simulink model "DNNCells_tSPMeA_BatteryPack_Passive100cellBal_RestCycler"  (R2024a)
settings: Solver=VariableStepAuto  StartTime=0.0  StopTime=1E7  RelTol=1e-3
undefined symbols (not defined in the file or in its folder): battery_builder_rtmsupport, gcbh
libraries: fl_lib x38, nesl_utility x36, simulink x26, BatteryLibrary_lib x6
(part 2 of 2)

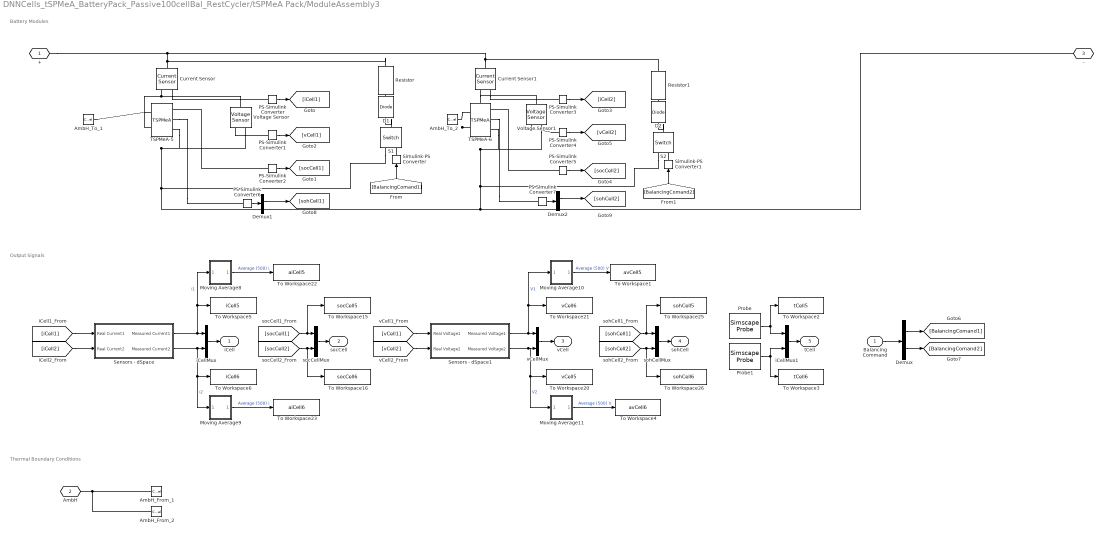
== system DNNCells_tSPMeA_BatteryPack_Passive100cellBal_RestCycler/tSPMeA Pack/ModuleAssembly3 ==
  note: Battery Modules
  note: Thermal Boundary Conditions
  note: Output Signals
  Balancing Command : Inport
  AmbH_From_1 : ConnectionLabel  Label=ambH_1
  AmbH_From_2 : ConnectionLabel  Label=ambH_2
  AmbH_To_1 : ConnectionLabel  Label=ambH_1
  AmbH_To_2 : ConnectionLabel  Label=ambH_2
  Current Sensor : fl_lib/Electrical/Electrical Sensors/Current Sensor
  Current Sensor1 : fl_lib/Electrical/Electrical Sensors/Current Sensor
  D1 : fl_lib/Electrical/Electrical Elements/Diode  Vf=0.6 V  Ron=0.3 Ohm  Goff=1e-8 1/Ohm  i_specify=off  i_priority=None  i=0 A  i_nominal_specify=off  i_nominal_value=1  i_nominal_unit=A  v_specify=off  v_priority=None  v=0 V  v_nominal_specify=off  v_nominal_value=1  v_nominal_unit=V
      settings: LogSimulationData=on
  D2 : fl_lib/Electrical/Electrical Elements/Diode  Vf=0.6 V  Ron=0.3 Ohm  Goff=1e-8 1/Ohm  i_specify=off  i_priority=None  i=0 A  i_nominal_specify=off  i_nominal_value=1  i_nominal_unit=A  v_specify=off  v_priority=None  v=0 V  v_nominal_specify=off  v_nominal_value=1  v_nominal_unit=V
      settings: LogSimulationData=on
  Demux : Demux  Outputs=2
  Demux1 : Demux
  Demux2 : Demux
  Moving Average10 : Subsystem
  Moving Average11 : Subsystem
  Moving Average8 : Subsystem
  Moving Average9 : Subsystem
  PS-Simulink Converter{,1..7} (8 alike) : nesl_utility/PS-Simulink Converter  PhysicalDomain=network_engine_domain  SubClassName=ps_output  LeftPortType=input  RightPortType=output  PseudoPeriodic=off  Frequencies=[]  VectorFormat=inherit  Unit=inherit  AffineConversion=off
  Probe : SimscapeProbe  BoundBlock=426  Variables={T}
  Probe1 : SimscapeProbe  BoundBlock=427  Variables={T}
  Resistor : fl_lib/Electrical/Electrical Elements/Resistor  R=0.001 Ohm  i_specify=off  i_priority=None  i=0 A  i_nominal_specify=off  i_nominal_value=1  i_nominal_unit=A  v_specify=off  v_priority=None  v=0 V  v_nominal_specify=off  v_nominal_value=1  v_nominal_unit=V
  Resistor1 : fl_lib/Electrical/Electrical Elements/Resistor  R=0.001 Ohm  i_specify=off  i_priority=None  i=0 A  i_nominal_specify=off  i_nominal_value=1  i_nominal_unit=A  v_specify=off  v_priority=None  v=0 V  v_nominal_specify=off  v_nominal_value=1  v_nominal_unit=V
  S1 : fl_lib/Electrical/Electrical Elements/Switch  R_closed=0.01 Ohm  G_open=1e-8 1/Ohm  Threshold=0.5  i_specify=off  i_priority=None  i=0 A  i_nominal_specify=off  i_nominal_value=1  i_nominal_unit=A  v_specify=off  v_priority=None  v=0 V  v_nominal_specify=off  v_nominal_value=1  v_nominal_unit=V
  S2 : fl_lib/Electrical/Electrical Elements/Switch  R_closed=0.01 Ohm  G_open=1e-8 1/Ohm  Threshold=0.5  i_specify=off  i_priority=None  i=0 A  i_nominal_specify=off  i_nominal_value=1  i_nominal_unit=A  v_specify=off  v_priority=None  v=0 V  v_nominal_specify=off  v_nominal_value=1  v_nominal_unit=V
  Sensors - dSpace : Subsystem
  Sensors - dSpace1 : Subsystem
  Simulink-PS Converter : nesl_utility/Simulink-PS Converter  PhysicalDomain=network_engine_domain  SubClassName=ps_input  LeftPortType=input  RightPortType=output  PseudoPeriodic=off  Frequencies=[]  NoiseDistribution=none  NoiseParameters=[]  Unit=1  AffineConversion=off  FilteringAndDerivatives=provide  SimscapeFilterOrder=1  InputFilterTimeConstant=0.001  UdotUserProvided=0
  Simulink-PS Converter1 : nesl_utility/Simulink-PS Converter  PhysicalDomain=network_engine_domain  SubClassName=ps_input  LeftPortType=input  RightPortType=output  PseudoPeriodic=off  Frequencies=[]  NoiseDistribution=none  NoiseParameters=[]  Unit=1  AffineConversion=off  FilteringAndDerivatives=provide  SimscapeFilterOrder=1  InputFilterTimeConstant=0.001  UdotUserProvided=0
  TSPMeA-5 : BatteryLibrary_lib/Models/TSPMeA  z0=cSoc5  T0=Ctemp5 K  eps_n0=0.25  Lf0=5E-3 um  Cn=4.9 A*hr  DnRef=3.3E-14 m^2/s  DpRef=4E-15 m^2/s  sigma_nRef=215 S/m  sigma_eRef=1.2 S/m  sigma_pRef=0.18 S/m  tr=0.2594  ce0=1000 mol/m^3  cn_max=33133 mol/m^3  cp_max=63104 mol/m^3  sn_max=0.9014  sn_min=0.0279  sp_max=0.9072  sp_min=0.2567  knRef=6.48E-7 A*m^(5/2)/mol^(3/2)  kpRef=3.42E-6 A*m^(5/2)/mol^(3/2)  Cp=110 J/K  Tref=298 K  Ea_kn=1 kJ/mol  Ea_kp=1 kJ/mol  Ea_Dn=75 kJ/mol  Ea_De=1.2 kJ/mol  Ea_Dp=10 kJ/mol  Ea_sigman=80 kJ/mol  Ea_sigmae=80 kJ/mol  Ea_sigmap=80 kJ/mol  Ea_ksei=1 kJ/mol  Ea_Dsei=1 kJ/mol  Ea_sigmasei=1 kJ/mol  Ea_kLi=1 kJ/mol  kseiRef=1E-12 m/s  DseiRef=2E-19 m^2/s  sigma_seiRef=5E-6 S/m  Msei=0.162 kg/mol  pho_sei=1690 kg/m^3  Usei=0 V  csei0=4541 mol/m^3  kLiRef=1E-11 m/s  ULi=0 V  MLi=6.94E-3 kg/mol  pho_Li=534 kg/m^3  Ln=85.2 um  Ls=12 um  Lp=75.6 um  Area_p=1027 cm^2  eps_s=0.47  eps_p=0.335  Rn=5.86 um  Rp=5.22 um  an=3.84E5 1/m  ap=3.82E5 1/m
      settings: InternalSimscapePortConfiguration="{\"Bottom\":[{\"id\":\"n\",\"label\":\"-\",\"type\":\"foundation.electrical.electrical\"}],\"Left\":[{\"id\":\"Hi\",\"label\":\"H\",\"type\":\"foundation.thermal.thermal\"}],\"Right\":[{\"id\":\"z\",\"label\":\"SoC\",\"type\":\"output\"},{\"id\":\"Lf_bar\",\"label\":\"sohF\",\"type\":\"output\"},{\"id\":\"SoH_Cn\",\"label\":\"sohC\",\"type\":\"output\"},{\"id\":\"pots\",\"label\":\"Pots\",\"type\":\"output\"}],\"Top\":[{\"id\":\"p\",\"label\":\"+\",\"type\":\"foundation.electrical.electrical\"}]}"
  TSPMeA-6 : BatteryLibrary_lib/Models/TSPMeA  z0=cSoc6  T0=Ctemp6 K  eps_n0=0.25  Lf0=5E-3 um  Cn=4.9 A*hr  DnRef=3.3E-14 m^2/s  DpRef=4E-15 m^2/s  sigma_nRef=215 S/m  sigma_eRef=1.2 S/m  sigma_pRef=0.18 S/m  tr=0.2594  ce0=1000 mol/m^3  cn_max=33133 mol/m^3  cp_max=63104 mol/m^3  sn_max=0.9014  sn_min=0.0279  sp_max=0.9072  sp_min=0.2567  knRef=6.48E-7 A*m^(5/2)/mol^(3/2)  kpRef=3.42E-6 A*m^(5/2)/mol^(3/2)  Cp=110 J/K  Tref=298 K  Ea_kn=1 kJ/mol  Ea_kp=1 kJ/mol  Ea_Dn=75 kJ/mol  Ea_De=1.2 kJ/mol  Ea_Dp=10 kJ/mol  Ea_sigman=80 kJ/mol  Ea_sigmae=80 kJ/mol  Ea_sigmap=80 kJ/mol  Ea_ksei=1 kJ/mol  Ea_Dsei=1 kJ/mol  Ea_sigmasei=1 kJ/mol  Ea_kLi=1 kJ/mol  kseiRef=1E-12 m/s  DseiRef=2E-19 m^2/s  sigma_seiRef=5E-6 S/m  Msei=0.162 kg/mol  pho_sei=1690 kg/m^3  Usei=0 V  csei0=4541 mol/m^3  kLiRef=1E-11 m/s  ULi=0 V  MLi=6.94E-3 kg/mol  pho_Li=534 kg/m^3  Ln=85.2 um  Ls=12 um  Lp=75.6 um  Area_p=1027 cm^2  eps_s=0.47  eps_p=0.335  Rn=5.86 um  Rp=5.22 um  an=3.84E5 1/m  ap=3.82E5 1/m
      settings: InternalSimscapePortConfiguration="{\"Bottom\":[{\"id\":\"n\",\"label\":\"-\",\"type\":\"foundation.electrical.electrical\"}],\"Left\":[{\"id\":\"Hi\",\"label\":\"H\",\"type\":\"foundation.thermal.thermal\"}],\"Right\":[{\"id\":\"z\",\"label\":\"SoC\",\"type\":\"output\"},{\"id\":\"Lf_bar\",\"label\":\"sohF\",\"type\":\"output\"},{\"id\":\"SoH_Cn\",\"label\":\"sohC\",\"type\":\"output\"},{\"id\":\"pots\",\"label\":\"Pots\",\"type\":\"output\"}],\"Top\":[{\"id\":\"p\",\"label\":\"+\",\"type\":\"foundation.electrical.electrical\"}]}"
  To Workspace1 : ToWorkspace  VariableName=avCell5  SampleTime=-1
  To Workspace15 : ToWorkspace  VariableName=socCell5  SampleTime=-1
  To Workspace16 : ToWorkspace  VariableName=socCell6  SampleTime=-1
  To Workspace2 : ToWorkspace  VariableName=tCell5  SampleTime=-1
  To Workspace20 : ToWorkspace  VariableName=vCell5  SampleTime=-1
  To Workspace21 : ToWorkspace  VariableName=vCell6  SampleTime=-1
  To Workspace22 : ToWorkspace  VariableName=aiCell5  SampleTime=-1
  To Workspace23 : ToWorkspace  VariableName=aiCell6  SampleTime=-1
  To Workspace25 : ToWorkspace  VariableName=sohCell5  SampleTime=-1
  To Workspace26 : ToWorkspace  VariableName=sohCell6  SampleTime=-1
  To Workspace3 : ToWorkspace  VariableName=tCell6  SampleTime=-1
  To Workspace4 : ToWorkspace  VariableName=avCell6  SampleTime=-1
  To Workspace5 : ToWorkspace  VariableName=iCell5  SampleTime=-1
  To Workspace6 : ToWorkspace  VariableName=iCell6  SampleTime=-1
  Voltage Sensor : fl_lib/Electrical/Electrical Sensors/Voltage Sensor
  Voltage Sensor1 : fl_lib/Electrical/Electrical Sensors/Voltage Sensor
  iCellMux : Mux  Inputs=2
  iCellMux1 : Mux  Inputs=2
  socCellMux : Mux  Inputs=2
  sohCellMux : Mux  Inputs=2
  vCellMux : Mux  Inputs=2
  + : PMIOPort  Side=Left
  AmbH : PMIOPort  Port=2  Side=Right  ConnectionType=Connection: foundation.thermal.thermal
  - : PMIOPort  Port=3  Side=Right
  iCell : Outport
  socCell : Outport  Port=2
  vCell : Outport  Port=3
  sohCell : Outport  Port=4
  tCell : Outport  Port=5
  wires:
  Balancing Command/1 -> Demux/1
  PS-Simulink Converter2/1 -> [socCell1]
  PS-Simulink Converter5/1 -> [socCell2]
  Demux/2 -> [BalancingComand2]
  PS-Simulink Converter/1 -> [iCell1]
  PS-Simulink Converter3/1 -> [iCell2]
  iCellMux/1 -> iCell/1
  vCellMux/1 -> vCell/1
  PS-Simulink Converter4/1 -> [vCell2]
  PS-Simulink Converter1/1 -> [vCell1]
  [BalancingComand2] -> Simulink-PS Converter1/1
  [BalancingComand1] -> Simulink-PS Converter/1
  socCellMux/1 -> socCell/1
  Demux/1 -> [BalancingComand1]
  PS-Simulink Converter7/1 -> Demux2/1
  Demux1/2 -> [sohCell1]
  sohCellMux/1 -> sohCell/1
  PS-Simulink Converter6/1 -> Demux1/1
  Demux2/2 -> [sohCell2]
  [socCell2] -> To Workspace16/1, socCellMux/2
  [socCell1] -> To Workspace15/1, socCellMux/1
  [sohCell1] -> To Workspace25/1, sohCellMux/1
  [sohCell2] -> To Workspace26/1, sohCellMux/2
  Probe1/1 -> To Workspace3/1, iCellMux1/2
  Probe/1 -> To Workspace2/1, iCellMux1/1
  iCellMux1/1 -> tCell/1
  Moving Average8/1(Out1) -> To Workspace22/1  "Average (500) i"
  Moving Average11/1(Out1) -> To Workspace4/1  "Average (500) V"
  Moving Average10/1(Out1) -> To Workspace1/1  "Average (500) V"
  Moving Average9/1(Out1) -> To Workspace23/1  "Average (500) i"
  [iCell1] -> Sensors - dSpace/1(Real Current1)
  [iCell2] -> Sensors - dSpace/2(Real Current2)
  Sensors - dSpace/1(Measured Current1) -> Moving Average8/1(Measured Current), To Workspace5/1, iCellMux/1  "i1"
  Sensors - dSpace/2(Measured Current2) -> Moving Average9/1(Measured Voltage), To Workspace6/1, iCellMux/2  "i2"
  [vCell1] -> Sensors - dSpace1/1(Real Voltage1)
  [vCell2] -> Sensors - dSpace1/2(Real Voltage2)
  Sensors - dSpace1/1(Measured Voltage1) -> Moving Average10/1(Measured Current), To Workspace21/1, vCellMux/1  "V1"
  Sensors - dSpace1/2(Measured Voltage2) -> Moving Average11/1(Measured Voltage), To Workspace20/1, vCellMux/2  "V2"
  connections:
  Current Sensor1/LConn1 -- Resistor1/LConn1 -- +/RConn1 -- Resistor/LConn1 -- Current Sensor/LConn1
  Voltage Sensor/RConn2 -- TSPMeA-5/RConn5 -- S1/RConn2 -- S2/RConn2 -- TSPMeA-6/RConn5 -- Voltage Sensor1/RConn2 -- -/RConn1
  TSPMeA-6/LConn2 -- Voltage Sensor1/LConn1 -- Current Sensor1/RConn2
  Voltage Sensor/LConn1 -- TSPMeA-5/LConn2 -- Current Sensor/RConn2
  AmbH_From_2/LConn1 -- AmbH/RConn1 -- AmbH_From_1/LConn1
  Simulink-PS Converter/RConn1 -- S1/RConn1
  D1/LConn1 -- Resistor/RConn1
  TSPMeA-6/LConn1 -- AmbH_To_2/LConn1
  PS-Simulink Converter4/LConn1 -- Voltage Sensor1/RConn1
  S1/LConn1 -- D1/RConn1
  Current Sensor/RConn1 -- PS-Simulink Converter/LConn1
  PS-Simulink Converter2/LConn1 -- TSPMeA-5/RConn1
  D2/LConn1 -- Resistor1/RConn1
  S2/LConn1 -- D2/RConn1
  TSPMeA-5/LConn1 -- AmbH_To_1/LConn1
  Voltage Sensor/RConn1 -- PS-Simulink Converter1/LConn1
  Simulink-PS Converter1/RConn1 -- S2/RConn1
  PS-Simulink Converter5/LConn1 -- TSPMeA-6/RConn1
  Current Sensor1/RConn1 -- PS-Simulink Converter3/LConn1
  TSPMeA-5/RConn3 -- PS-Simulink Converter6/LConn1
  TSPMeA-6/RConn3 -- PS-Simulink Converter7/LConn1

== system DNNCells_tSPMeA_BatteryPack_Passive100cellBal_RestCycler/tSPMeA Pack/ModuleAssembly1/Moving Average ==
  Measured Current : Inport
  Product : Product  Inputs=*/
  Sum of Elements : Sum  Inputs=+
  Tapped Delay : simulink/Discrete/Tapped Delay  vinit=0.0  samptime=-1  NumDelays=499  DelayOrder=Oldest  includeCurrent=off
  Vector Concatenate : Concatenate
  Width : Width
  Out1 : Outport
  wires:
  Sum of Elements/1 -> Product/1
  Vector Concatenate/1 -> Width/1, Sum of Elements/1
  Product/1 -> Out1/1
  Tapped Delay/1 -> Vector Concatenate/2
  Measured Current/1 -> Tapped Delay/1, Vector Concatenate/1
  Width/1 -> Product/2

== system DNNCells_tSPMeA_BatteryPack_Passive100cellBal_RestCycler/tSPMeA Pack/ModuleAssembly1/Moving Average1 ==
  Measured Voltage : Inport
  Product : Product  Inputs=*/
  Sum of Elements : Sum  Inputs=+
  Tapped Delay : simulink/Discrete/Tapped Delay  vinit=0.0  samptime=-1  NumDelays=499  DelayOrder=Oldest  includeCurrent=off
  Vector Concatenate : Concatenate
  Width : Width
  Out1 : Outport
  wires:
  Sum of Elements/1 -> Product/1
  Vector Concatenate/1 -> Width/1, Sum of Elements/1
  Product/1 -> Out1/1
  Tapped Delay/1 -> Vector Concatenate/2
  Measured Voltage/1 -> Tapped Delay/1, Vector Concatenate/1
  Width/1 -> Product/2

== system DNNCells_tSPMeA_BatteryPack_Passive100cellBal_RestCycler/tSPMeA Pack/ModuleAssembly1/Moving Average2 ==
  Measured Current : Inport
  Product : Product  Inputs=*/
  Sum of Elements : Sum  Inputs=+
  Tapped Delay : simulink/Discrete/Tapped Delay  vinit=0.0  samptime=-1  NumDelays=499  DelayOrder=Oldest  includeCurrent=off
  Vector Concatenate : Concatenate
  Width : Width
  Out1 : Outport
  wires:
  Sum of Elements/1 -> Product/1
  Vector Concatenate/1 -> Width/1, Sum of Elements/1
  Product/1 -> Out1/1
  Tapped Delay/1 -> Vector Concatenate/2
  Measured Current/1 -> Tapped Delay/1, Vector Concatenate/1
  Width/1 -> Product/2

== system DNNCells_tSPMeA_BatteryPack_Passive100cellBal_RestCycler/tSPMeA Pack/ModuleAssembly1/Moving Average3 ==
  Measured Voltage : Inport
  Product : Product  Inputs=*/
  Sum of Elements : Sum  Inputs=+
  Tapped Delay : simulink/Discrete/Tapped Delay  vinit=0.0  samptime=-1  NumDelays=499  DelayOrder=Oldest  includeCurrent=off
  Vector Concatenate : Concatenate
  Width : Width
  Out1 : Outport
  wires:
  Sum of Elements/1 -> Product/1
  Vector Concatenate/1 -> Width/1, Sum of Elements/1
  Product/1 -> Out1/1
  Tapped Delay/1 -> Vector Concatenate/2
  Measured Voltage/1 -> Tapped Delay/1, Vector Concatenate/1
  Width/1 -> Product/2

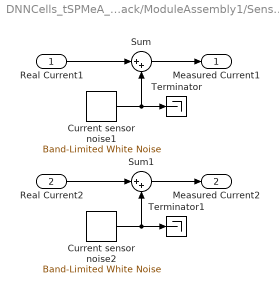
== system DNNCells_tSPMeA_BatteryPack_Passive100cellBal_RestCycler/tSPMeA Pack/ModuleAssembly1/Sensors - dSpace ==
  Real Current1 : Inport
  Real Current2 : Inport  Port=2
  Current sensor noise1 : simulink/Sources/Band-Limited White Noise  Cov=1e-3  Ts=1  seed=1
  Current sensor noise2 : simulink/Sources/Band-Limited White Noise  Cov=1e-3  Ts=1  seed=23341
  Sum : Sum  Inputs=|++
  Sum1 : Sum  Inputs=|++
  Terminator : Terminator
  Terminator1 : Terminator
  Measured Current1 : Outport
  Measured Current2 : Outport  Port=2
  wires:
  Current sensor noise2/1 -> Terminator1/1, Sum1/2
  Current sensor noise1/1 -> Sum/2, Terminator/1
  Real Current1/1 -> Sum/1
  Sum1/1 -> Measured Current2/1
  Sum/1 -> Measured Current1/1
  Real Current2/1 -> Sum1/1

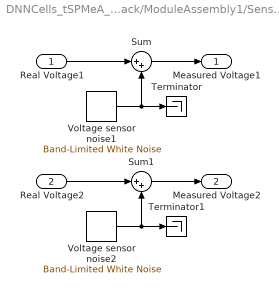
== system DNNCells_tSPMeA_BatteryPack_Passive100cellBal_RestCycler/tSPMeA Pack/ModuleAssembly1/Sensors - dSpace1 ==
  Real Voltage1 : Inport
  Real Voltage2 : Inport  Port=2
  Sum : Sum  Inputs=|++
  Sum1 : Sum  Inputs=|++
  Terminator : Terminator
  Terminator1 : Terminator
  Voltage sensor noise1 : simulink/Sources/Band-Limited White Noise  Cov=1e-3  Ts=1  seed=1
  Voltage sensor noise2 : simulink/Sources/Band-Limited White Noise  Cov=1e-3  Ts=1  seed=23341
  Measured Voltage1 : Outport
  Measured Voltage2 : Outport  Port=2
  wires:
  Voltage sensor noise2/1 -> Terminator1/1, Sum1/2
  Voltage sensor noise1/1 -> Sum/2, Terminator/1
  Real Voltage1/1 -> Sum/1
  Sum1/1 -> Measured Voltage2/1
  Sum/1 -> Measured Voltage1/1
  Real Voltage2/1 -> Sum1/1

== system DNNCells_tSPMeA_BatteryPack_Passive100cellBal_RestCycler/tSPMeA Pack/ModuleAssembly2/Moving Average4 ==
  Measured Current : Inport
  Product : Product  Inputs=*/
  Sum of Elements : Sum  Inputs=+
  Tapped Delay : simulink/Discrete/Tapped Delay  vinit=0.0  samptime=-1  NumDelays=499  DelayOrder=Oldest  includeCurrent=off
  Vector Concatenate : Concatenate
  Width : Width
  Out1 : Outport
  wires:
  Sum of Elements/1 -> Product/1
  Vector Concatenate/1 -> Width/1, Sum of Elements/1
  Product/1 -> Out1/1
  Tapped Delay/1 -> Vector Concatenate/2
  Measured Current/1 -> Tapped Delay/1, Vector Concatenate/1
  Width/1 -> Product/2

== system DNNCells_tSPMeA_BatteryPack_Passive100cellBal_RestCycler/tSPMeA Pack/ModuleAssembly2/Moving Average5 ==
  Measured Voltage : Inport
  Product : Product  Inputs=*/
  Sum of Elements : Sum  Inputs=+
  Tapped Delay : simulink/Discrete/Tapped Delay  vinit=0.0  samptime=-1  NumDelays=499  DelayOrder=Oldest  includeCurrent=off
  Vector Concatenate : Concatenate
  Width : Width
  Out1 : Outport
  wires:
  Sum of Elements/1 -> Product/1
  Vector Concatenate/1 -> Width/1, Sum of Elements/1
  Product/1 -> Out1/1
  Tapped Delay/1 -> Vector Concatenate/2
  Measured Voltage/1 -> Tapped Delay/1, Vector Concatenate/1
  Width/1 -> Product/2

== system DNNCells_tSPMeA_BatteryPack_Passive100cellBal_RestCycler/tSPMeA Pack/ModuleAssembly2/Moving Average6 ==
  Measured Current : Inport
  Product : Product  Inputs=*/
  Sum of Elements : Sum  Inputs=+
  Tapped Delay : simulink/Discrete/Tapped Delay  vinit=0.0  samptime=-1  NumDelays=499  DelayOrder=Oldest  includeCurrent=off
  Vector Concatenate : Concatenate
  Width : Width
  Out1 : Outport
  wires:
  Sum of Elements/1 -> Product/1
  Vector Concatenate/1 -> Width/1, Sum of Elements/1
  Product/1 -> Out1/1
  Tapped Delay/1 -> Vector Concatenate/2
  Measured Current/1 -> Tapped Delay/1, Vector Concatenate/1
  Width/1 -> Product/2

== system DNNCells_tSPMeA_BatteryPack_Passive100cellBal_RestCycler/tSPMeA Pack/ModuleAssembly2/Moving Average7 ==
  Measured Voltage : Inport
  Product : Product  Inputs=*/
  Sum of Elements : Sum  Inputs=+
  Tapped Delay : simulink/Discrete/Tapped Delay  vinit=0.0  samptime=-1  NumDelays=499  DelayOrder=Oldest  includeCurrent=off
  Vector Concatenate : Concatenate
  Width : Width
  Out1 : Outport
  wires:
  Sum of Elements/1 -> Product/1
  Vector Concatenate/1 -> Width/1, Sum of Elements/1
  Product/1 -> Out1/1
  Tapped Delay/1 -> Vector Concatenate/2
  Measured Voltage/1 -> Tapped Delay/1, Vector Concatenate/1
  Width/1 -> Product/2

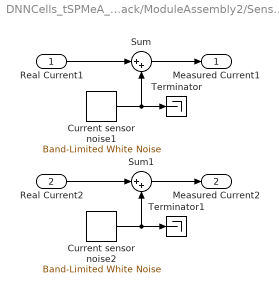
== system DNNCells_tSPMeA_BatteryPack_Passive100cellBal_RestCycler/tSPMeA Pack/ModuleAssembly2/Sensors - dSpace ==
  Real Current1 : Inport
  Real Current2 : Inport  Port=2
  Current sensor noise1 : simulink/Sources/Band-Limited White Noise  Cov=1e-3  Ts=1  seed=1
  Current sensor noise2 : simulink/Sources/Band-Limited White Noise  Cov=1e-3  Ts=1  seed=23341
  Sum : Sum  Inputs=|++
  Sum1 : Sum  Inputs=|++
  Terminator : Terminator
  Terminator1 : Terminator
  Measured Current1 : Outport
  Measured Current2 : Outport  Port=2
  wires:
  Current sensor noise2/1 -> Terminator1/1, Sum1/2
  Current sensor noise1/1 -> Sum/2, Terminator/1
  Real Current1/1 -> Sum/1
  Sum1/1 -> Measured Current2/1
  Sum/1 -> Measured Current1/1
  Real Current2/1 -> Sum1/1

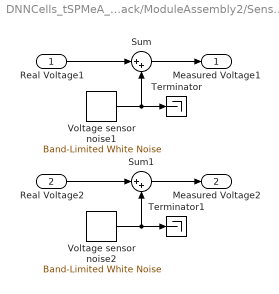
== system DNNCells_tSPMeA_BatteryPack_Passive100cellBal_RestCycler/tSPMeA Pack/ModuleAssembly2/Sensors - dSpace1 ==
  Real Voltage1 : Inport
  Real Voltage2 : Inport  Port=2
  Sum : Sum  Inputs=|++
  Sum1 : Sum  Inputs=|++
  Terminator : Terminator
  Terminator1 : Terminator
  Voltage sensor noise1 : simulink/Sources/Band-Limited White Noise  Cov=1e-3  Ts=1  seed=1
  Voltage sensor noise2 : simulink/Sources/Band-Limited White Noise  Cov=1e-3  Ts=1  seed=23341
  Measured Voltage1 : Outport
  Measured Voltage2 : Outport  Port=2
  wires:
  Voltage sensor noise2/1 -> Terminator1/1, Sum1/2
  Voltage sensor noise1/1 -> Sum/2, Terminator/1
  Real Voltage1/1 -> Sum/1
  Sum1/1 -> Measured Voltage2/1
  Sum/1 -> Measured Voltage1/1
  Real Voltage2/1 -> Sum1/1

== system DNNCells_tSPMeA_BatteryPack_Passive100cellBal_RestCycler/tSPMeA Pack/ModuleAssembly3/Moving Average10 ==
  Measured Current : Inport
  Product : Product  Inputs=*/
  Sum of Elements : Sum  Inputs=+
  Tapped Delay : simulink/Discrete/Tapped Delay  vinit=0.0  samptime=-1  NumDelays=499  DelayOrder=Oldest  includeCurrent=off
  Vector Concatenate : Concatenate
  Width : Width
  Out1 : Outport
  wires:
  Sum of Elements/1 -> Product/1
  Vector Concatenate/1 -> Width/1, Sum of Elements/1
  Product/1 -> Out1/1
  Tapped Delay/1 -> Vector Concatenate/2
  Measured Current/1 -> Tapped Delay/1, Vector Concatenate/1
  Width/1 -> Product/2

== system DNNCells_tSPMeA_BatteryPack_Passive100cellBal_RestCycler/tSPMeA Pack/ModuleAssembly3/Moving Average11 ==
  Measured Voltage : Inport
  Product : Product  Inputs=*/
  Sum of Elements : Sum  Inputs=+
  Tapped Delay : simulink/Discrete/Tapped Delay  vinit=0.0  samptime=-1  NumDelays=499  DelayOrder=Oldest  includeCurrent=off
  Vector Concatenate : Concatenate
  Width : Width
  Out1 : Outport
  wires:
  Sum of Elements/1 -> Product/1
  Vector Concatenate/1 -> Width/1, Sum of Elements/1
  Product/1 -> Out1/1
  Tapped Delay/1 -> Vector Concatenate/2
  Measured Voltage/1 -> Tapped Delay/1, Vector Concatenate/1
  Width/1 -> Product/2

== system DNNCells_tSPMeA_BatteryPack_Passive100cellBal_RestCycler/tSPMeA Pack/ModuleAssembly3/Moving Average8 ==
  Measured Current : Inport
  Product : Product  Inputs=*/
  Sum of Elements : Sum  Inputs=+
  Tapped Delay : simulink/Discrete/Tapped Delay  vinit=0.0  samptime=-1  NumDelays=499  DelayOrder=Oldest  includeCurrent=off
  Vector Concatenate : Concatenate
  Width : Width
  Out1 : Outport
  wires:
  Sum of Elements/1 -> Product/1
  Vector Concatenate/1 -> Width/1, Sum of Elements/1
  Product/1 -> Out1/1
  Tapped Delay/1 -> Vector Concatenate/2
  Measured Current/1 -> Tapped Delay/1, Vector Concatenate/1
  Width/1 -> Product/2

== system DNNCells_tSPMeA_BatteryPack_Passive100cellBal_RestCycler/tSPMeA Pack/ModuleAssembly3/Moving Average9 ==
  Measured Voltage : Inport
  Product : Product  Inputs=*/
  Sum of Elements : Sum  Inputs=+
  Tapped Delay : simulink/Discrete/Tapped Delay  vinit=0.0  samptime=-1  NumDelays=499  DelayOrder=Oldest  includeCurrent=off
  Vector Concatenate : Concatenate
  Width : Width
  Out1 : Outport
  wires:
  Sum of Elements/1 -> Product/1
  Vector Concatenate/1 -> Width/1, Sum of Elements/1
  Product/1 -> Out1/1
  Tapped Delay/1 -> Vector Concatenate/2
  Measured Voltage/1 -> Tapped Delay/1, Vector Concatenate/1
  Width/1 -> Product/2

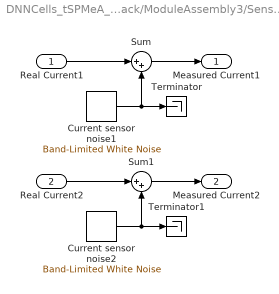
== system DNNCells_tSPMeA_BatteryPack_Passive100cellBal_RestCycler/tSPMeA Pack/ModuleAssembly3/Sensors - dSpace ==
  Real Current1 : Inport
  Real Current2 : Inport  Port=2
  Current sensor noise1 : simulink/Sources/Band-Limited White Noise  Cov=1e-3  Ts=1  seed=1
  Current sensor noise2 : simulink/Sources/Band-Limited White Noise  Cov=1e-3  Ts=1  seed=23341
  Sum : Sum  Inputs=|++
  Sum1 : Sum  Inputs=|++
  Terminator : Terminator
  Terminator1 : Terminator
  Measured Current1 : Outport
  Measured Current2 : Outport  Port=2
  wires:
  Current sensor noise2/1 -> Terminator1/1, Sum1/2
  Current sensor noise1/1 -> Sum/2, Terminator/1
  Real Current1/1 -> Sum/1
  Sum1/1 -> Measured Current2/1
  Sum/1 -> Measured Current1/1
  Real Current2/1 -> Sum1/1

== system DNNCells_tSPMeA_BatteryPack_Passive100cellBal_RestCycler/tSPMeA Pack/ModuleAssembly3/Sensors - dSpace1 ==
  Real Voltage1 : Inport
  Real Voltage2 : Inport  Port=2
  Sum : Sum  Inputs=|++
  Sum1 : Sum  Inputs=|++
  Terminator : Terminator
  Terminator1 : Terminator
  Voltage sensor noise1 : simulink/Sources/Band-Limited White Noise  Cov=1e-3  Ts=1  seed=1
  Voltage sensor noise2 : simulink/Sources/Band-Limited White Noise  Cov=1e-3  Ts=1  seed=23341
  Measured Voltage1 : Outport
  Measured Voltage2 : Outport  Port=2
  wires:
  Voltage sensor noise2/1 -> Terminator1/1, Sum1/2
  Voltage sensor noise1/1 -> Sum/2, Terminator/1
  Real Voltage1/1 -> Sum/1
  Sum1/1 -> Measured Voltage2/1
  Sum/1 -> Measured Voltage1/1
  Real Voltage2/1 -> Sum1/1

== matlab function DNNCells_tSPMeA_BatteryPack_Passive100cellBal_RestCycler/MATLAB Function ==
  data: SOCvec input; command output
function command = fcn(SOCvec)

command = zeros([1 length(SOCvec)]);

for i = 1:length(SOCvec)
    if SOCvec(i) >= 0.8
        command(i) = 1;
    end
end

if max(SOCvec)-min(SOCvec) <= 0.02
    command = zeros([1 length(SOCvec)]);
end
